simulink model "with_glideslope_and_flare"  (R2021b)
settings: Solver=VariableStepAuto  StartTime=0.0  StopTime=145  RelTol=1e-3
values from neighbouring files (symbols this model uses):
  h_flare = 45    [chapter8.m]
  SS_long_lo = ss(SS_lo.A(long_states,long_states), SS_lo.B(long_states,long_inputs), SS_lo.C(long_outputs,long_states), SS_lo.D(long_outputs,long_inputs))    [FindF16Dynamics.m]    (also in chapter5.m; chapter6.m; chapter7.m; chapter8.m = ss(SS_lo.A(long_states,long_states),                  SS_lo.)
  tau = 2.867    [chapter8.m]
  trim_state_lin = trim_state_lo    [FindF16Dynamics.m]    (also in chapter5.m; chapter6.m; chapter7.m; chapter8.m)
libraries: slpidlib x4, simulink x1
settings Model: Creator=User  LastModifiedBy=User

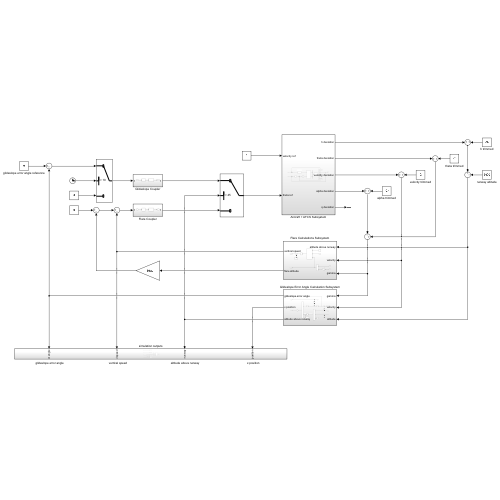
[thumbnail: Simulink's stored preview of the top-level diagram]
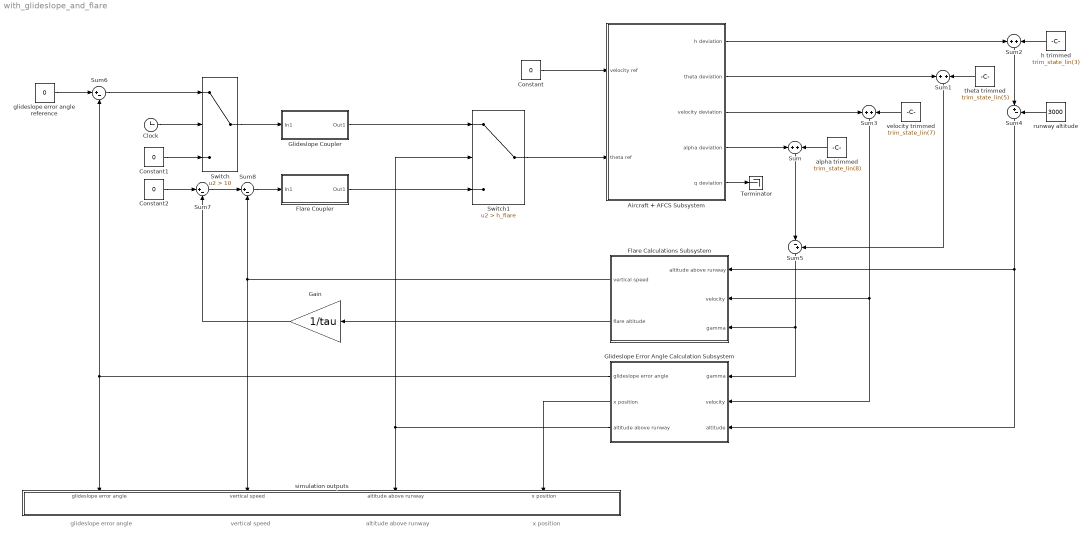
== system with_glideslope_and_flare ==
  note: x position
  note: altitude above runway
  note: vertical speed
  note: glideslope error angle
  Aircraft + AFCS Subsystem : Subsystem
  Clock : Clock
  Constant : Constant  Value=0
  Constant1 : Constant  Value=0
  Constant2 : Constant  Value=0
  Flare Calculations Subsystem : Subsystem
  Flare Coupler : Subsystem
  Gain : Gain  Gain=1/tau
  Glideslope Coupler : Subsystem
  Glideslope Error Angle Calculation Subsystem : Subsystem
  Sum{,1..3} (4 alike) : Sum  Inputs=+|+
  Sum{4,6..8} (4 alike) : Sum  Inputs=|+-
  Sum5 : Sum  Inputs=|-+
  Switch : Switch  Criteria=u2 > Threshold  Threshold=10
  Switch1 : Switch  Criteria=u2 > Threshold  Threshold=h_flare
  Terminator : Terminator
  alpha trimmed : Constant  Value=trim_state_lin(8)
  glideslope error angle reference : Constant  Value=0
  h trimmed : Constant  Value=trim_state_lin(3)
  runway altitude : Constant  Value=3000
  simulation outputs : Subsystem
  theta trimmed : Constant  Value=trim_state_lin(5)
  velocity trimmed : Constant  Value=trim_state_lin(7)
  wires:
  Constant/1 -> Aircraft + AFCS Subsystem/1(velocity ref)
  Aircraft + AFCS Subsystem/1(h deviation) -> Sum2/1
  Aircraft + AFCS Subsystem/2(theta deviation) -> Sum1/1
  Aircraft + AFCS Subsystem/3(velocity deviation) -> Sum3/1
  Aircraft + AFCS Subsystem/5(q deviation) -> Terminator/1
  Aircraft + AFCS Subsystem/4(alpha deviation) -> Sum/1
  alpha trimmed/1 -> Sum/2
  velocity trimmed/1 -> Sum3/2
  theta trimmed/1 -> Sum1/2
  h trimmed/1 -> Sum2/2
  Sum/1 -> Sum5/1
  Sum1/1 -> Sum5/2
  runway altitude/1 -> Sum4/2
  Sum2/1 -> Sum4/1
  Sum4/1 -> Glideslope Error Angle Calculation Subsystem/3(altitude), Flare Calculations Subsystem/1(altitude above runway)
  Switch/1 -> Glideslope Coupler/1(In1)
  Sum5/1 -> Glideslope Error Angle Calculation Subsystem/1(gamma), Flare Calculations Subsystem/3(gamma)
  Glideslope Error Angle Calculation Subsystem/1(glideslope error angle) -> simulation outputs/1(glideslope error angle), Sum6/2
  Clock/1 -> Switch/2
  Constant1/1 -> Switch/3
  Sum6/1 -> Switch/1
  glideslope error angle reference/1 -> Sum6/1
  Glideslope Coupler/1(Out1) -> Switch1/1
  Glideslope Error Angle Calculation Subsystem/2(x position) -> simulation outputs/4(x position)
  Switch1/1 -> Aircraft + AFCS Subsystem/2(theta ref)
  Flare Coupler/1(Out1) -> Switch1/3
  Glideslope Error Angle Calculation Subsystem/3(altitude above runway) -> Switch1/2, simulation outputs/3(altitude above runway)
  Constant2/1 -> Sum7/1
  Sum7/1 -> Sum8/1
  Sum8/1 -> Flare Coupler/1(In1)
  Flare Calculations Subsystem/1(vertical speed) -> Sum8/2, simulation outputs/2(vertical speed)
  Flare Calculations Subsystem/2(flare altitude) -> Gain/1
  Sum3/1 -> Glideslope Error Angle Calculation Subsystem/2(velocity), Flare Calculations Subsystem/2(velocity)
  Gain/1 -> Sum7/2

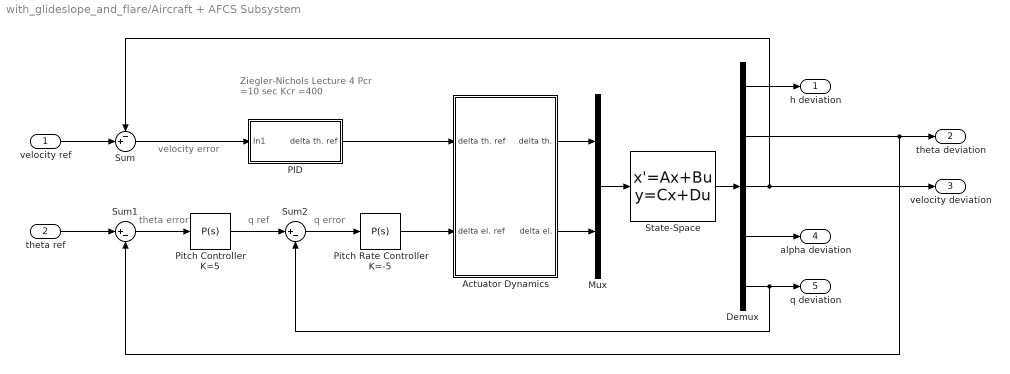
== system with_glideslope_and_flare/Aircraft + AFCS Subsystem ==
  note: q error
  note: q ref
  note: theta error
  note: velocity error
  note: Ziegler-Nichols Lecture 4
      | Pcr =10 sec
      | Kcr =400
  velocity ref : Inport
  theta ref : Inport  Port=2
  Actuator Dynamics : Subsystem
  Demux : Demux  Outputs=5
  Mux : Mux  Inputs=2
  PID : Subsystem
  Pitch Controller K=5 : slpidlib/PID Controller  Controller=P  Form=Parallel  TimeDomain=Continuous-time  UseExternalTs=off  SampleTime=-1  IntegratorMethod=Forward Euler  FilterMethod=Forward Euler  ControllerParametersSource=internal  P=5  I=3.43247113169158  D=5.95190934365968  UseFilter=on  N=361.191549741391  TunerSelectOption=Transfer Function Based (PID Tuner App)  InitialConditionSource=internal  InitialConditionForIntegrator=0  InitialConditionForFilter=0  DifferentiatorICPrevScaledInput=0  ExternalReset=none  TrackingMode=off  Kt=1  LimitOutput=off  SatLimitsSource=internal  UpperSaturationLimit=inf  LowerSaturationLimit=-inf  LinearizeAsGain=on  AntiWindupMode=none  Kb=1  POutMin=[]  POutMax=[]  IOutMin=[]  IOutMax=[]  DOutMin=[]  DOutMax=[]  NOutMin=[]  NOutMax=[]  SumOutMin=[]  SumOutMax=[]  SaturationOutMin=[]  SaturationOutMax=[]  PParamMin=[]  PParamMax=[]  IParamMin=[]  IParamMax=[]  DParamMin=[]  DParamMax=[]  NParamMin=[]  NParamMax=[]  KbParamMin=[]  KbParamMax=[]  KtParamMin=[]  KtParamMax=[]  KbOutMin=[]  KbOutMax=[]  KtOutMin=[]  KtOutMax=[]  IntegratorOutMin=[]  IntegratorOutMax=[]  FilterOutMin=[]  FilterOutMax=[]  SumI1OutMin=[]  SumI1OutMax=[]  SumI2OutMin=[]  SumI2OutMax=[]  SumI3OutMin=[]  SumI3OutMax=[]  SumI4OutMin=[]  SumI4OutMax=[]  SumDOutMin=[]  SumDOutMax=[]  DifferentiatorOutMin=[]  DifferentiatorOutMax=[]  FilterDiffOutCoefMin=[]  FilterDiffOutCoefMax=[]  ReciprocalOutMin=[]  ReciprocalOutMax=[]  SumDenOutMin=[]  SumDenOutMax=[]  SumNumOutMin=[]  SumNumOutMax=[]  DivideOutMin=[]  DivideOutMax=[]  UdiffTsProdOutMin=[]  UdiffTsProdOutMax=[]  NTsProdOutMin=[]  NTsProdOutMax=[]  UintegralTsProdOutMin=[]  UintegralTsProdOutMax=[]  UngainTsProdOutMin=[]  UngainTsProdOutMax=[]  IntegratorContinuousStateAttributes=''  IntegratorStateMustResolveToSignalObject=off  IntegratorRTWStateStorageClass=Auto  FilterContinuousStateAttributes=''  FilterStateMustResolveToSignalObject=off  FilterRTWStateStorageClass=Auto  ParallelPVariant=InternalParameters  IdealPVariant=Disabled  IVariant=Disabled  DVariant=Disabled  IntegratorVariant=Disabled  SatVariant=Disabled  AWVariant=Disabled  PCopyVariant=Disabled  TRVariant=Disabled  FdbkBlocksVariant=Forward  IdealPFdbkVariant=Disabled  SatFdbkVariant=Disabled  DerivativeFilterVariant=Disabled  NVariant=Disabled  NCopyVariant=Disabled_SignalSpec  FilterICVariant=Disabled  IntegratorICVariant=Disabled  ExternalResetVariant=Disabled  TRSumVariant=Passthrough  SumFdbkVariant=Disabled  SumVariant=Passthrough_P  TsampFilterVariant=InternalTs  TsampNgainVariant=Passthrough  TsampIntegralVariant=Disabled_SignalSpec  ExternalSaturationOutDataTypeStr=Inherit: Same as second input
  Pitch Rate Controller K=-5 : slpidlib/PID Controller  Controller=P  Form=Parallel  TimeDomain=Continuous-time  UseExternalTs=off  SampleTime=-1  IntegratorMethod=Forward Euler  FilterMethod=Forward Euler  ControllerParametersSource=internal  P=-5  I=-0.00395211653661635  D=-0.0895160383616166  UseFilter=on  N=1.43348723146542  TunerSelectOption=Transfer Function Based (PID Tuner App)  InitialConditionSource=internal  InitialConditionForIntegrator=0  InitialConditionForFilter=0  DifferentiatorICPrevScaledInput=0  ExternalReset=none  TrackingMode=off  Kt=1  LimitOutput=off  SatLimitsSource=internal  UpperSaturationLimit=inf  LowerSaturationLimit=-inf  LinearizeAsGain=on  AntiWindupMode=none  Kb=1  POutMin=[]  POutMax=[]  IOutMin=[]  IOutMax=[]  DOutMin=[]  DOutMax=[]  NOutMin=[]  NOutMax=[]  SumOutMin=[]  SumOutMax=[]  SaturationOutMin=[]  SaturationOutMax=[]  PParamMin=[]  PParamMax=[]  IParamMin=[]  IParamMax=[]  DParamMin=[]  DParamMax=[]  NParamMin=[]  NParamMax=[]  KbParamMin=[]  KbParamMax=[]  KtParamMin=[]  KtParamMax=[]  KbOutMin=[]  KbOutMax=[]  KtOutMin=[]  KtOutMax=[]  IntegratorOutMin=[]  IntegratorOutMax=[]  FilterOutMin=[]  FilterOutMax=[]  SumI1OutMin=[]  SumI1OutMax=[]  SumI2OutMin=[]  SumI2OutMax=[]  SumI3OutMin=[]  SumI3OutMax=[]  SumI4OutMin=[]  SumI4OutMax=[]  SumDOutMin=[]  SumDOutMax=[]  DifferentiatorOutMin=[]  DifferentiatorOutMax=[]  FilterDiffOutCoefMin=[]  FilterDiffOutCoefMax=[]  ReciprocalOutMin=[]  ReciprocalOutMax=[]  SumDenOutMin=[]  SumDenOutMax=[]  SumNumOutMin=[]  SumNumOutMax=[]  DivideOutMin=[]  DivideOutMax=[]  UdiffTsProdOutMin=[]  UdiffTsProdOutMax=[]  NTsProdOutMin=[]  NTsProdOutMax=[]  UintegralTsProdOutMin=[]  UintegralTsProdOutMax=[]  UngainTsProdOutMin=[]  UngainTsProdOutMax=[]  IntegratorContinuousStateAttributes=''  IntegratorStateMustResolveToSignalObject=off  IntegratorRTWStateStorageClass=Auto  FilterContinuousStateAttributes=''  FilterStateMustResolveToSignalObject=off  FilterRTWStateStorageClass=Auto  ParallelPVariant=InternalParameters  IdealPVariant=Disabled  IVariant=Disabled  DVariant=Disabled  IntegratorVariant=Disabled  SatVariant=Disabled  AWVariant=Disabled  PCopyVariant=Disabled  TRVariant=Disabled  FdbkBlocksVariant=Forward  IdealPFdbkVariant=Disabled  SatFdbkVariant=Disabled  DerivativeFilterVariant=Disabled  NVariant=Disabled  NCopyVariant=Disabled_SignalSpec  FilterICVariant=Disabled  IntegratorICVariant=Disabled  ExternalResetVariant=Disabled  TRSumVariant=Passthrough  SumFdbkVariant=Disabled  SumVariant=Passthrough_P  TsampFilterVariant=InternalTs  TsampNgainVariant=Passthrough  TsampIntegralVariant=Disabled_SignalSpec  ExternalSaturationOutDataTypeStr=Inherit: Same as second input
  State-Space : StateSpace  A=SS_long_lo.A  B=SS_long_lo.B  C=SS_long_lo.C  D=SS_long_lo.D  InitialCondition=0
  Sum : Sum  Inputs=-+|
  Sum1 : Sum  Inputs=|+-
  Sum2 : Sum  Inputs=|+-
  h deviation : Outport
  theta deviation : Outport  Port=2
  velocity deviation : Outport  Port=3
  alpha deviation : Outport  Port=4
  q deviation : Outport  Port=5
  wires:
  velocity ref/1 -> Sum/2
  Demux/3 -> velocity deviation/1, Sum/1
  State-Space/1 -> Demux/1
  Demux/4 -> alpha deviation/1
  Demux/5 -> q deviation/1, Sum2/2
  Demux/2 -> theta deviation/1, Sum1/2
  Demux/1 -> h deviation/1
  Mux/1 -> State-Space/1
  Actuator Dynamics/1(delta th.) -> Mux/1
  Actuator Dynamics/2(delta el.) -> Mux/2
  theta ref/1 -> Sum1/1
  Pitch Rate Controller K=-5/1 -> Actuator Dynamics/2(delta el. ref)
  Sum1/1 -> Pitch Controller K=5/1
  Pitch Controller K=5/1 -> Sum2/1
  Sum2/1 -> Pitch Rate Controller K=-5/1
  Sum/1 -> PID/1(In1)
  PID/1(delta th. ref) -> Actuator Dynamics/1(delta th. ref)

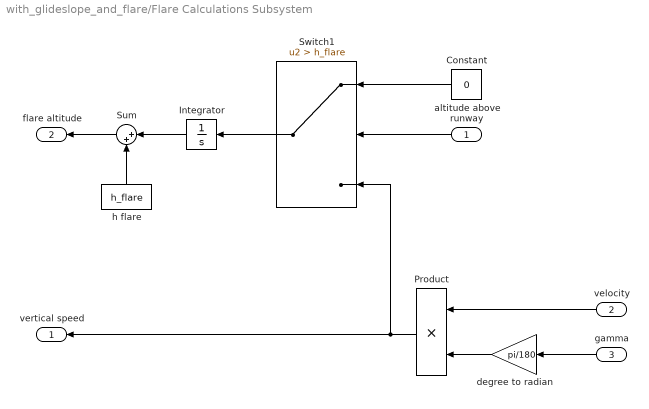
== system with_glideslope_and_flare/Flare Calculations Subsystem ==
  altitude above runway : Inport
  velocity : Inport  Port=2
  gamma : Inport  Port=3
  Constant : Constant  Value=0
  Integrator : Integrator
  Product : Product
  Sum : Sum  Inputs=|++
  Switch1 : Switch  Criteria=u2 > Threshold  Threshold=h_flare
  degree to radian : Gain  Gain=pi/180
  h flare : Constant  Value=h_flare
  vertical speed : Outport
  flare altitude : Outport  Port=2
  wires:
  gamma/1 -> degree to radian/1
  degree to radian/1 -> Product/2
  velocity/1 -> Product/1
  Product/1 -> vertical speed/1, Switch1/3
  altitude above runway/1 -> Switch1/2
  Constant/1 -> Switch1/1
  Switch1/1 -> Integrator/1
  Sum/1 -> flare altitude/1
  Integrator/1 -> Sum/1
  h flare/1 -> Sum/2

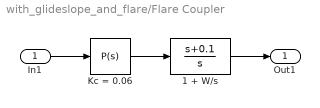
== system with_glideslope_and_flare/Flare Coupler ==
  In1 : Inport
  1 + W/s : TransferFcn  Numerator=[1 0.1]  Denominator=[1 0]
  Kc = 0.06 : slpidlib/PID Controller  Controller=P  Form=Parallel  TimeDomain=Continuous-time  UseExternalTs=off  SampleTime=-1  IntegratorMethod=Forward Euler  FilterMethod=Forward Euler  ControllerParametersSource=internal  P=0.06  I=0  D=0  UseFilter=on  N=100  TunerSelectOption=Transfer Function Based (PID Tuner App)  InitialConditionSource=internal  InitialConditionForIntegrator=0  InitialConditionForFilter=0  DifferentiatorICPrevScaledInput=0  ExternalReset=none  TrackingMode=off  Kt=1  LimitOutput=off  SatLimitsSource=internal  UpperSaturationLimit=inf  LowerSaturationLimit=-inf  LinearizeAsGain=on  AntiWindupMode=none  Kb=1  POutMin=[]  POutMax=[]  IOutMin=[]  IOutMax=[]  DOutMin=[]  DOutMax=[]  NOutMin=[]  NOutMax=[]  SumOutMin=[]  SumOutMax=[]  SaturationOutMin=[]  SaturationOutMax=[]  PParamMin=[]  PParamMax=[]  IParamMin=[]  IParamMax=[]  DParamMin=[]  DParamMax=[]  NParamMin=[]  NParamMax=[]  KbParamMin=[]  KbParamMax=[]  KtParamMin=[]  KtParamMax=[]  KbOutMin=[]  KbOutMax=[]  KtOutMin=[]  KtOutMax=[]  IntegratorOutMin=[]  IntegratorOutMax=[]  FilterOutMin=[]  FilterOutMax=[]  SumI1OutMin=[]  SumI1OutMax=[]  SumI2OutMin=[]  SumI2OutMax=[]  SumI3OutMin=[]  SumI3OutMax=[]  SumI4OutMin=[]  SumI4OutMax=[]  SumDOutMin=[]  SumDOutMax=[]  DifferentiatorOutMin=[]  DifferentiatorOutMax=[]  FilterDiffOutCoefMin=[]  FilterDiffOutCoefMax=[]  ReciprocalOutMin=[]  ReciprocalOutMax=[]  SumDenOutMin=[]  SumDenOutMax=[]  SumNumOutMin=[]  SumNumOutMax=[]  DivideOutMin=[]  DivideOutMax=[]  UdiffTsProdOutMin=[]  UdiffTsProdOutMax=[]  NTsProdOutMin=[]  NTsProdOutMax=[]  UintegralTsProdOutMin=[]  UintegralTsProdOutMax=[]  UngainTsProdOutMin=[]  UngainTsProdOutMax=[]  IntegratorContinuousStateAttributes=''  IntegratorStateMustResolveToSignalObject=off  IntegratorRTWStateStorageClass=Auto  FilterContinuousStateAttributes=''  FilterStateMustResolveToSignalObject=off  FilterRTWStateStorageClass=Auto  ParallelPVariant=InternalParameters  IdealPVariant=Disabled  IVariant=Disabled  DVariant=Disabled  IntegratorVariant=Disabled  SatVariant=Disabled  AWVariant=Disabled  PCopyVariant=Disabled  TRVariant=Disabled  FdbkBlocksVariant=Forward  IdealPFdbkVariant=Disabled  SatFdbkVariant=Disabled  DerivativeFilterVariant=Disabled  NVariant=Disabled  NCopyVariant=Disabled_SignalSpec  FilterICVariant=Disabled  IntegratorICVariant=Disabled  ExternalResetVariant=Disabled  TRSumVariant=Passthrough  SumFdbkVariant=Disabled  SumVariant=Passthrough_P  TsampFilterVariant=InternalTs  TsampNgainVariant=Passthrough  TsampIntegralVariant=Disabled_SignalSpec  ExternalSaturationOutDataTypeStr=Inherit: Same as second input
  Out1 : Outport
  wires:
  In1/1 -> Kc = 0.06/1
  Kc = 0.06/1 -> 1 + W/s/1
  1 + W/s/1 -> Out1/1

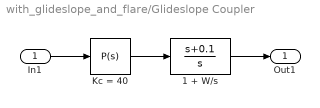
== system with_glideslope_and_flare/Glideslope Coupler ==
  In1 : Inport
  1 + W/s : TransferFcn  Numerator=[1 0.1]  Denominator=[1 0]
  Kc = 40 : slpidlib/PID Controller  Controller=P  Form=Parallel  TimeDomain=Continuous-time  UseExternalTs=off  SampleTime=-1  IntegratorMethod=Forward Euler  FilterMethod=Forward Euler  ControllerParametersSource=internal  P=40  I=0  D=0  UseFilter=on  N=100  TunerSelectOption=Transfer Function Based (PID Tuner App)  InitialConditionSource=internal  InitialConditionForIntegrator=0  InitialConditionForFilter=0  DifferentiatorICPrevScaledInput=0  ExternalReset=none  TrackingMode=off  Kt=1  LimitOutput=off  SatLimitsSource=internal  UpperSaturationLimit=inf  LowerSaturationLimit=-inf  LinearizeAsGain=on  AntiWindupMode=none  Kb=1  POutMin=[]  POutMax=[]  IOutMin=[]  IOutMax=[]  DOutMin=[]  DOutMax=[]  NOutMin=[]  NOutMax=[]  SumOutMin=[]  SumOutMax=[]  SaturationOutMin=[]  SaturationOutMax=[]  PParamMin=[]  PParamMax=[]  IParamMin=[]  IParamMax=[]  DParamMin=[]  DParamMax=[]  NParamMin=[]  NParamMax=[]  KbParamMin=[]  KbParamMax=[]  KtParamMin=[]  KtParamMax=[]  KbOutMin=[]  KbOutMax=[]  KtOutMin=[]  KtOutMax=[]  IntegratorOutMin=[]  IntegratorOutMax=[]  FilterOutMin=[]  FilterOutMax=[]  SumI1OutMin=[]  SumI1OutMax=[]  SumI2OutMin=[]  SumI2OutMax=[]  SumI3OutMin=[]  SumI3OutMax=[]  SumI4OutMin=[]  SumI4OutMax=[]  SumDOutMin=[]  SumDOutMax=[]  DifferentiatorOutMin=[]  DifferentiatorOutMax=[]  FilterDiffOutCoefMin=[]  FilterDiffOutCoefMax=[]  ReciprocalOutMin=[]  ReciprocalOutMax=[]  SumDenOutMin=[]  SumDenOutMax=[]  SumNumOutMin=[]  SumNumOutMax=[]  DivideOutMin=[]  DivideOutMax=[]  UdiffTsProdOutMin=[]  UdiffTsProdOutMax=[]  NTsProdOutMin=[]  NTsProdOutMax=[]  UintegralTsProdOutMin=[]  UintegralTsProdOutMax=[]  UngainTsProdOutMin=[]  UngainTsProdOutMax=[]  IntegratorContinuousStateAttributes=''  IntegratorStateMustResolveToSignalObject=off  IntegratorRTWStateStorageClass=Auto  FilterContinuousStateAttributes=''  FilterStateMustResolveToSignalObject=off  FilterRTWStateStorageClass=Auto  ParallelPVariant=InternalParameters  IdealPVariant=Disabled  IVariant=Disabled  DVariant=Disabled  IntegratorVariant=Disabled  SatVariant=Disabled  AWVariant=Disabled  PCopyVariant=Disabled  TRVariant=Disabled  FdbkBlocksVariant=Forward  IdealPFdbkVariant=Disabled  SatFdbkVariant=Disabled  DerivativeFilterVariant=Disabled  NVariant=Disabled  NCopyVariant=Disabled_SignalSpec  FilterICVariant=Disabled  IntegratorICVariant=Disabled  ExternalResetVariant=Disabled  TRSumVariant=Passthrough  SumFdbkVariant=Disabled  SumVariant=Passthrough_P  TsampFilterVariant=InternalTs  TsampNgainVariant=Passthrough  TsampIntegralVariant=Disabled_SignalSpec  ExternalSaturationOutDataTypeStr=Inherit: Same as second input
  Out1 : Outport
  wires:
  In1/1 -> Kc = 40/1
  Kc = 40/1 -> 1 + W/s/1
  1 + W/s/1 -> Out1/1

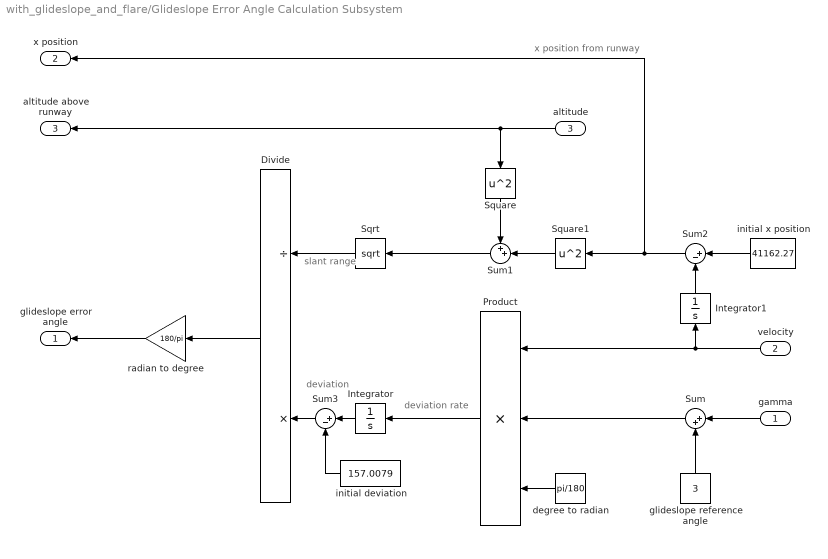
== system with_glideslope_and_flare/Glideslope Error Angle Calculation Subsystem ==
  note: slant range
  note: x position from runway
  note: deviation
  note: deviation rate
  gamma : Inport
  velocity : Inport  Port=2
  altitude : Inport  Port=3
  Divide : Product  Inputs=/*
  Integrator : Integrator
  Integrator1 : Integrator
  Product : Product  Inputs=3
  Sqrt : Sqrt  SaturateOnIntegerOverflow=on
  Square : Math  Operator=square  SaturateOnIntegerOverflow=on
  Square1 : Math  Operator=square  SaturateOnIntegerOverflow=on
  Sum : Sum  Inputs=|++
  Sum1 : Sum  Inputs=++|
  Sum2 : Sum  Inputs=|+-
  Sum3 : Sum  Inputs=|+-
  degree to radian : Constant  Value=pi/180
  glideslope reference angle : Constant  Value=3
  initial deviation : Constant  Value=157.0079
  initial x position : Constant  Value=41162.27
  radian to degree : Gain  Gain=180/pi
  glideslope error angle : Outport
  x position : Outport  Port=2
  altitude above runway : Outport  Port=3
  wires:
  altitude/1 -> Square/1, altitude above runway/1
  degree to radian/1 -> Product/3
  velocity/1 -> Product/1, Integrator1/1
  gamma/1 -> Sum/1
  glideslope reference angle/1 -> Sum/2
  Sum/1 -> Product/2
  Product/1 -> Integrator/1
  Integrator/1 -> Sum3/1
  Divide/1 -> radian to degree/1
  radian to degree/1 -> glideslope error angle/1
  Sqrt/1 -> Divide/1
  Sum1/1 -> Sqrt/1
  Square/1 -> Sum1/1
  Integrator1/1 -> Sum2/2
  Sum2/1 -> Square1/1, x position/1
  Square1/1 -> Sum1/2
  initial x position/1 -> Sum2/1
  Sum3/1 -> Divide/2
  initial deviation/1 -> Sum3/2

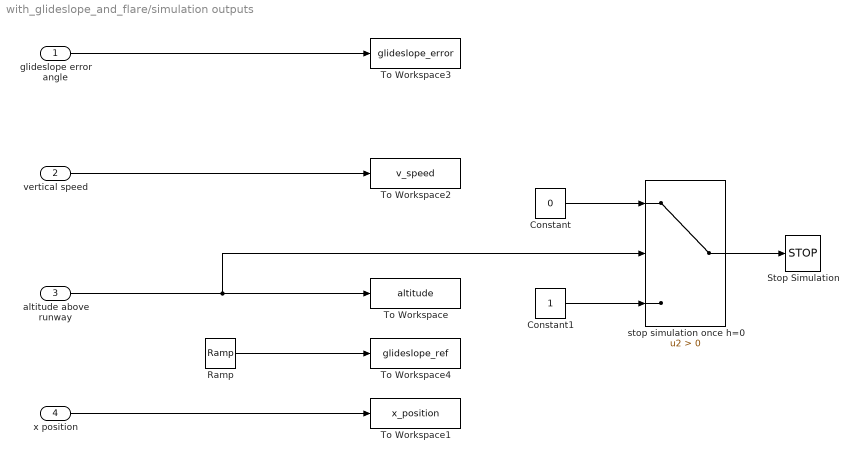
== system with_glideslope_and_flare/simulation outputs ==
  glideslope error angle : Inport
  vertical speed : Inport  Port=2
  altitude above runway : Inport  Port=3
  x position : Inport  Port=4
  Constant : Constant  Value=0
  Constant1 : Constant
  Ramp : simulink/Sources/Ramp  slope=-trim_state_lin(7)*3*pi/180  start=10  InitialOutput=2000
  Stop Simulation : Stop
  To Workspace : ToWorkspace  VariableName=altitude  SaveFormat=Structure With Time  SampleTime=-1
  To Workspace1 : ToWorkspace  VariableName=x_position  SaveFormat=Structure With Time  SampleTime=-1
  To Workspace2 : ToWorkspace  VariableName=v_speed  SaveFormat=Structure With Time  SampleTime=-1
  To Workspace3 : ToWorkspace  VariableName=glideslope_error  SaveFormat=Structure With Time  SampleTime=-1
  To Workspace4 : ToWorkspace  VariableName=glideslope_ref  SaveFormat=Structure With Time  SampleTime=-1
  stop simulation once h=0 : Switch  Criteria=u2 > Threshold
  wires:
  altitude above runway/1 -> To Workspace/1, stop simulation once h=0/2
  x position/1 -> To Workspace1/1
  vertical speed/1 -> To Workspace2/1
  glideslope error angle/1 -> To Workspace3/1
  stop simulation once h=0/1 -> Stop Simulation/1
  Constant1/1 -> stop simulation once h=0/3
  Constant/1 -> stop simulation once h=0/1
  Ramp/1 -> To Workspace4/1

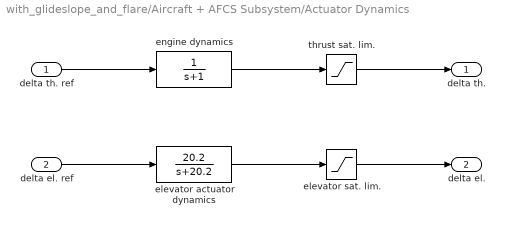
== system with_glideslope_and_flare/Aircraft + AFCS Subsystem/Actuator Dynamics ==
  delta th. ref : Inport
  delta el. ref : Inport  Port=2
  elevator actuator dynamics : TransferFcn  Numerator=[20.2]  Denominator=[1 20.2]
  elevator sat. lim. : Saturate  UpperLimit=29.1891  LowerLimit=-20.8109
  engine dynamics : TransferFcn  Denominator=[1 1]
  thrust sat. lim. : Saturate  UpperLimit=16173.1835  LowerLimit=-1826.8165
  delta th. : Outport
  delta el. : Outport  Port=2
  wires:
  delta el. ref/1 -> elevator actuator dynamics/1
  elevator actuator dynamics/1 -> elevator sat. lim./1
  elevator sat. lim./1 -> delta el./1
  thrust sat. lim./1 -> delta th./1
  engine dynamics/1 -> thrust sat. lim./1
  delta th. ref/1 -> engine dynamics/1

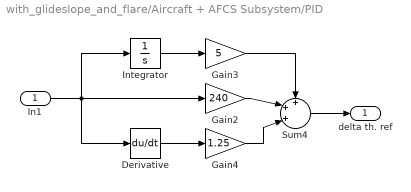
== system with_glideslope_and_flare/Aircraft + AFCS Subsystem/PID ==
  In1 : Inport
  Derivative : Derivative
  Gain2 : Gain  Gain=240
  Gain3 : Gain  Gain=5
  Gain4 : Gain  Gain=1.25
  Integrator : Integrator
  Sum4 : Sum  Inputs=+++|
  delta th. ref : Outport
  wires:
  Gain4/1 -> Sum4/3
  Gain3/1 -> Sum4/1
  Derivative/1 -> Gain4/1
  Integrator/1 -> Gain3/1
  Sum4/1 -> delta th. ref/1
  In1/1 -> Integrator/1, Derivative/1, Gain2/1
  Gain2/1 -> Sum4/2
